simulink model "model"  (R2022b)
settings: Solver=ode3  StartTime=0.0  StopTime=1  FixedStep=0.0005  RelTol=1e-3
values from neighbouring files (symbols this model uses):
  a21 = 1/2/m * x30^2 * FemP1/FemP2^2 * exp(-x10/FemP2)    [init.m]    (also in proj.m)
  a23 = -1/m * x30 * FemP1/FemP2 * exp(-x10/FemP2)    [init.m]    (also in proj.m)
  a31 = 1/f1 * exp(x10/f2) * (ki*u10 + ci - x30)    [init.m]    (also in proj.m)
  a33 = -f2/f1 * exp(x10/f2)    [init.m]    (also in proj.m)
  b31 = ki * f2/f1 * exp(x10/f2)    [init.m]    (also in proj.m)
  g = 9.81    [init.m]    (also in proj.m)
  xd = d-bd    [init.m]    (also in proj.m)
settings Model: Creator=TheZl  LastModifiedBy=TheZl

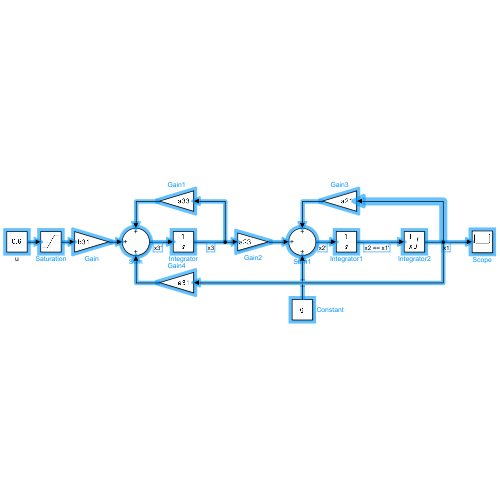
[thumbnail: Simulink's stored preview of the top-level diagram]
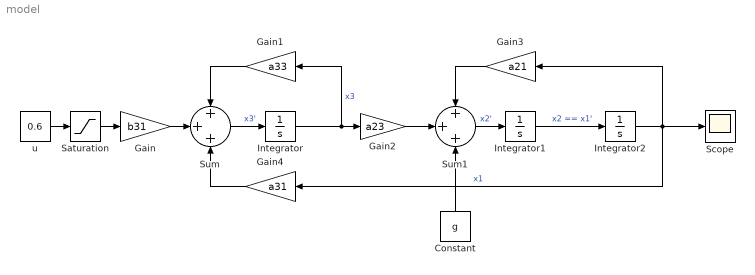
== system model ==
  Constant : Constant  Value=g
  Gain : Gain  Gain=b31
  Gain1 : Gain  Gain=a33
  Gain2 : Gain  Gain=a23
  Gain3 : Gain  Gain=a21
  Gain4 : Gain  Gain=a31
  Integrator : Integrator
  Integrator1 : Integrator
  Integrator2 : Integrator  InitialCondition=xd  LimitOutput=on  UpperSaturationLimit=xd  LowerSaturationLimit=0
  Saturation : Saturate  UpperLimit=1  LowerLimit=0
  Scope : Scope
  Sum : Sum  Inputs=+++
  Sum1 : Sum  Inputs=+++
  u : Constant  Value=0.6
  wires:
  Gain/1 -> Sum/2
  Sum/1 -> Integrator/1  "x3'"
  Gain1/1 -> Sum/1
  Integrator/1 -> Gain1/1, Gain2/1  "x3"
  Gain2/1 -> Sum1/2
  Gain3/1 -> Sum1/1
  Sum1/1 -> Integrator1/1  "x2'"
  Integrator1/1 -> Integrator2/1  "x2 == x1'"
  Gain4/1 -> Sum/3
  Integrator2/1 -> Scope/1, Gain4/1, Gain3/1  "x1"
  Constant/1 -> Sum1/3
  Saturation/1 -> Gain/1
  u/1 -> Saturation/1
